simulink model "MPC_Extended_Plant_Simulink"  (R2024a)
settings: Solver=ode4  StartTime=0.0  StopTime=20  FixedStep=1e-3  RelTol=1e-3
values from neighbouring files (symbols this model uses):
  init =     [P1.mat]    (also in P2.mat; P3.mat)
  input =     [P1.mat]    (also in P2.mat; P3.mat)
  par =     [P1.mat]    (also in P2.mat; P3.mat)
  Ts = 0.01    [MPC_Extended_Plant.m]    (also in P1.mat; P2.mat; P3.mat)
  V_ref = 16.6666666667    [P1.mat]    (also in P2.mat; P3.mat)
undefined symbols (not defined in the file or in its folder): data
libraries: simulink x8
(part 1 of 2)
settings Model: Creator=bshyrokau  LastModifiedBy=lbsch
settings SolverCC: AlgebraicLoopSolver=TrustRegion
settings DataIOCC: SaveOutput=off  SignalLogging=off  DSMLogging=off  SaveTime=off  ReturnWorkspaceOutputs=off
settings OptimizationCC: ReuseModelBlockBuffer=off  LifeSpan=inf
settings DebuggingCC: UnconnectedInputMsg=warning  UnconnectedOutputMsg=warning  UnconnectedLineMsg=warning  AllowSymbolicDim=off  SFUnexpectedBacktrackingDiag=warning  SFNoUnconditionalDefaultTransitionDiag=warning  SFExecutionAtInitializationDiag=none  ArithmeticOperatorsInVariantConditions=warning
settings ModelReferenceCC: EnableRefExpFcnMdlSchedulingChecks=on  PropagateSignalLabelsOutOfModel=off
settings SFSimCC: SimUseLocalCustomCode=off  CustomCodeUndefinedFunction=UseInterfaceOnly
settings RTWCC: RTWUseLocalCustomCode=off  GPUComputeCapability=3.5  DLArmComputeVersion=19.05
settings CodeAppCC: StateflowObjectComments=on
settings GRTTargetCC: TargetLangStandard=C89/C90 (ANSI)
settings ConfigComp: CovMetricSettings=dw  CovSaveCumulativeToWorkspaceVar=on  CovSaveSingleToWorkspaceVar=on  CovExternalEMLEnable=off
settings SimscapeCC: SimscapeNormalizeSystem=off
settings ConfigurationSet: Description=SimMechanics 2G

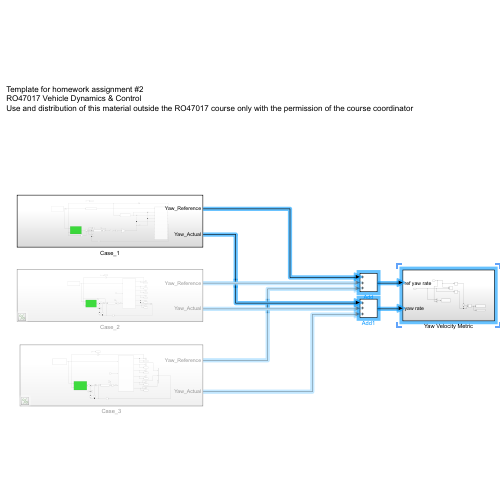
[thumbnail: Simulink's stored preview of the top-level diagram]
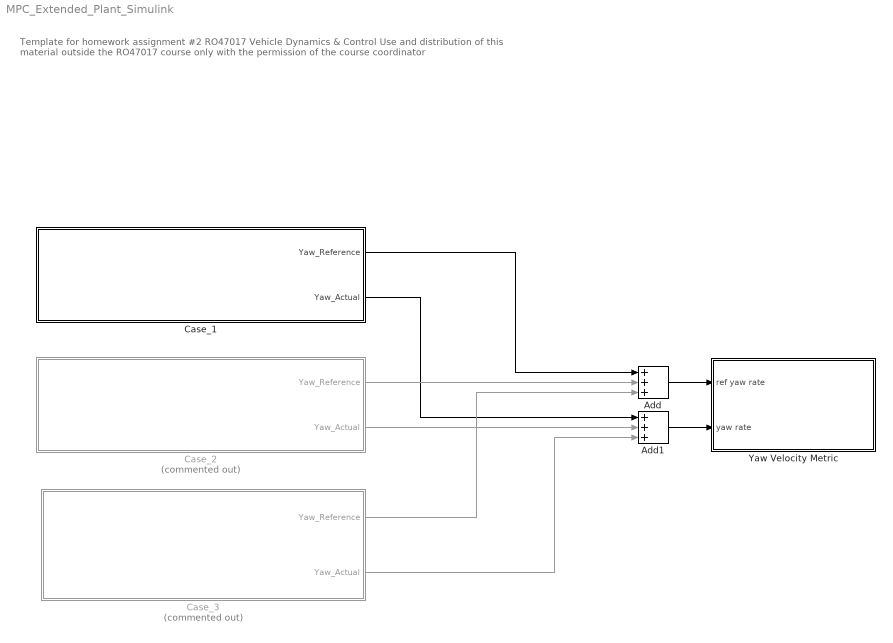
== system MPC_Extended_Plant_Simulink ==
  note: Template for homework assignment #2
      | RO47017 Vehicle Dynamics & Control
      | Use and distribution of this material outside the RO47017 course only with the permission of the course coordinator
  Add : Sum  Inputs=3
  Add1 : Sum  Inputs=3
  Case_1 : Subsystem
  Case_2 : Subsystem  Commented=on
  Case_3 : Subsystem  Commented=on
  Yaw Velocity Metric : Subsystem
  wires:
  Case_1/1(Yaw_Reference) -> Add/1
  Add/1 -> Yaw Velocity Metric/1(ref yaw rate)
  Case_1/2(Yaw_Actual) -> Add1/1
  Case_3/2(Yaw_Actual) -> Add1/3
  Case_3/1(Yaw_Reference) -> Add/3
  Case_2/2(Yaw_Actual) -> Add1/2
  Case_2/1(Yaw_Reference) -> Add/2
  Add1/1 -> Yaw Velocity Metric/2(yaw rate)

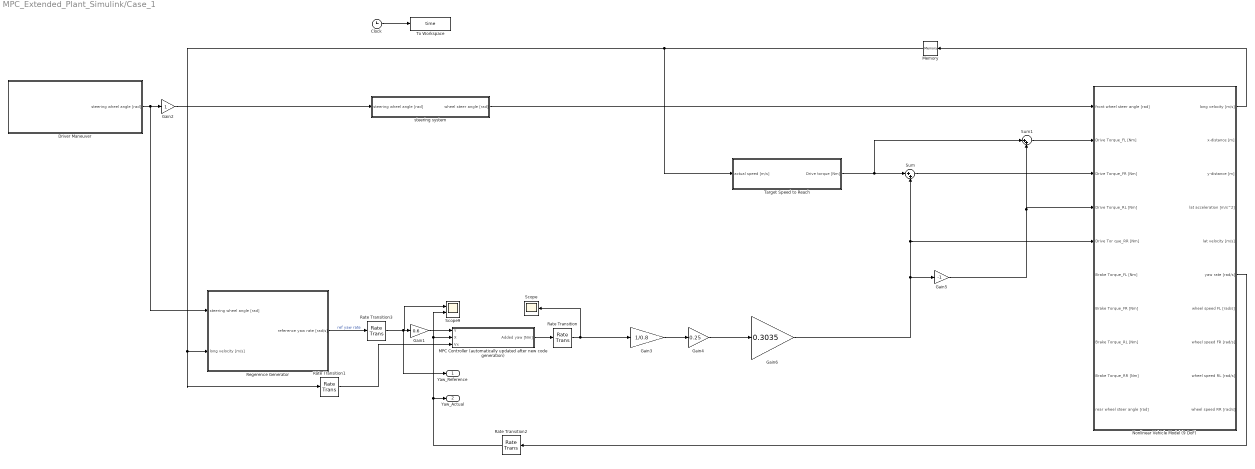
== system MPC_Extended_Plant_Simulink/Case_1 ==
  Clock : Clock
  Driver Maneuver : Subsystem
  Gain1 : Gain  Gain=0.6
  Gain2 : Gain
  Gain3 : Gain  Gain=1/0.8
  Gain4 : Gain  Gain=0.25
  Gain5 : Gain  Gain=-1
  Gain6 : Gain  Gain=0.3035
  MPC Controller (automatically updated after new code generation) : Subsystem
  Memory : Memory  InitialCondition=V_ref
  Nonlinear Vehicle Model (9 DoF) : Subsystem
      mask help: Simulink:masks:GenSFuncDesc_MD
      mask Help: eval('feval(''rtwprivate'',''rtwhelpview'',''rtw_sfcn_block'')');
  Rate Transition : RateTransition
  Rate Transition1 : RateTransition  InitialCondition=V_ref  OutPortSampleTime=Ts
  Rate Transition2 : RateTransition  OutPortSampleTime=Ts
  Rate Transition3 : RateTransition  OutPortSampleTime=Ts
  Regerence Generator : Subsystem
  Scope : Scope
  Scope9 : Scope  NumInputPorts=2
  Sum : Sum  Inputs=|++
  Sum1 : Sum  Inputs=|++
  Target Speed to Reach : Subsystem
  To Workspace : ToWorkspace  VariableName=time  SampleTime=-1
  steering system : Subsystem
  Yaw_Reference : Outport
  Yaw_Actual : Outport  Port=2
  wires:
  MPC Controller (automatically updated after new code generation)/1(Added yaw [Nm]) -> Rate Transition/1
  Gain1/1 -> MPC Controller (automatically updated after new code generation)/1(Y)
  Rate Transition2/1 -> Yaw_Actual/1, Scope9/2, MPC Controller (automatically updated after new code generation)/2(X)
  Rate Transition3/1 -> Yaw_Reference/1, Gain1/1, Scope9/1
  Clock/1 -> To Workspace/1
  Rate Transition1/1 -> MPC Controller (automatically updated after new code generation)/3(Vx)
  Rate Transition/1 -> Scope/1, Gain3/1
  Regerence Generator/1(reference yaw rate [rad/s]) -> Rate Transition3/1  "ref yaw rate"
  Driver Maneuver/1(steering wheel angle [rad]) -> Regerence Generator/1(steering wheel angle [rad]), Gain2/1
  Gain2/1 -> steering system/1(steering wheel angle [rad])
  steering system/1(wheel steer angle [rad]) -> Nonlinear Vehicle Model (9 DoF)/1(front wheel steer angle [rad])
  Gain6/1 -> Gain5/1, Nonlinear Vehicle Model (9 DoF)/5(Drive Tor	que_RR [Nm]), Sum/2
  Gain4/1 -> Gain6/1
  Gain3/1 -> Gain4/1
  Gain5/1 -> Nonlinear Vehicle Model (9 DoF)/4(Drive Torque_RL [Nm]), Sum1/2
  Nonlinear Vehicle Model (9 DoF)/6(yaw rate [rad/s]) -> Rate Transition2/1
  Sum/1 -> Nonlinear Vehicle Model (9 DoF)/3(Drive Torque_FR [Nm])
  Target Speed to Reach/1(Drive torque [Nm]) -> Sum1/1, Sum/1
  Sum1/1 -> Nonlinear Vehicle Model (9 DoF)/2(Drive Torque_FL [Nm])
  Memory/1 -> Rate Transition1/1, Regerence Generator/2(long velocity [m/s]), Target Speed to Reach/1(actual speed [m/s])
  Nonlinear Vehicle Model (9 DoF)/1(long velocity [m/s]) -> Memory/1

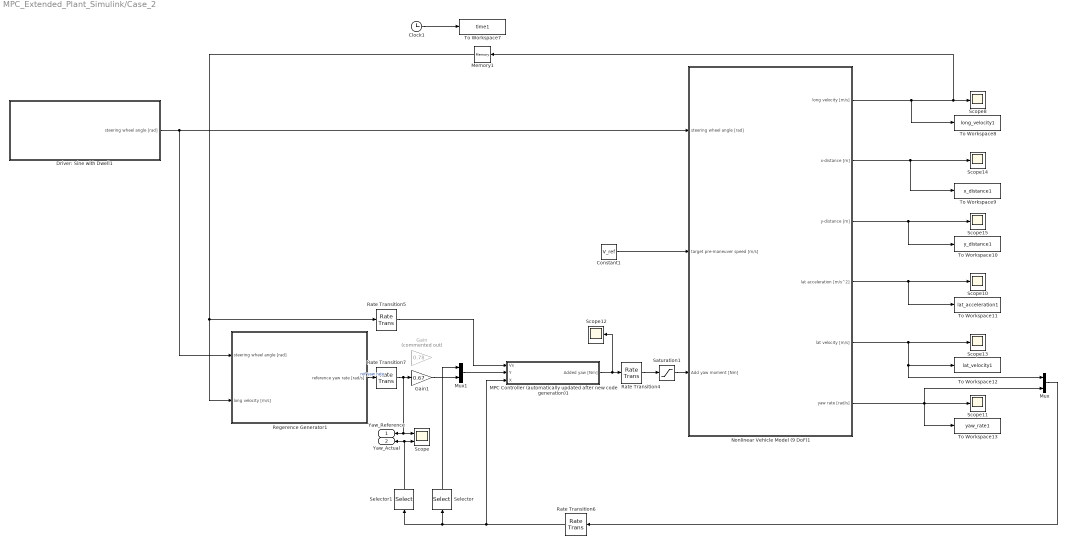
== system MPC_Extended_Plant_Simulink/Case_2 ==
  Clock1 : Clock
  Constant1 : Constant  Value=V_ref
  Driver: Sine with Dwell1 : Subsystem
  Gain : Gain  Commented=on  Gain=0.78
  Gain1 : Gain  Gain=0.67
  MPC Controller (automatically updated after new code generation)1 : Subsystem
  Memory1 : Memory  InitialCondition=V_ref
  Mux : Mux  Inputs=2
  Mux1 : Mux  Inputs=2
  Nonlinear Vehicle Model (9 DoF)1 : Subsystem
      mask help: Simulink:masks:GenSFuncDesc_MD
      mask Help: eval('feval(''rtwprivate'',''rtwhelpview'',''rtw_sfcn_block'')');
  Rate Transition4 : RateTransition
  Rate Transition5 : RateTransition  InitialCondition=V_ref  OutPortSampleTime=Ts
  Rate Transition6 : RateTransition  InitialCondition=[0 0]  OutPortSampleTime=Ts
  Rate Transition7 : RateTransition  OutPortSampleTime=Ts
  Regerence Generator1 : Subsystem
  Saturation1 : Saturate  UpperLimit=10000  LowerLimit=-10000
  Scope : Scope  NumInputPorts=2
  Scope{8,10..15} (7 alike) : Scope
  Selector : Selector  InputPortWidth=2  IndexOptions=Index vector (dialog)  Indices=1  OutputSizes=1
  Selector1 : Selector  InputPortWidth=2  IndexOptions=Index vector (dialog)  Indices=2  OutputSizes=1
  To Workspace10 : ToWorkspace  VariableName=y_distance1  SampleTime=-1
  To Workspace11 : ToWorkspace  VariableName=lat_acceleration1  SampleTime=-1
  To Workspace12 : ToWorkspace  VariableName=lat_velocity1  SampleTime=-1
  To Workspace13 : ToWorkspace  VariableName=yaw_rate1  SampleTime=-1
  To Workspace7 : ToWorkspace  VariableName=time1  SampleTime=-1
  To Workspace8 : ToWorkspace  VariableName=long_velocity1  SampleTime=-1
  To Workspace9 : ToWorkspace  VariableName=x_distance1  SampleTime=-1
  Yaw_Reference : Outport
  Yaw_Actual : Outport  Port=2
  wires:
  Rate Transition4/1 -> Saturation1/1
  Nonlinear Vehicle Model (9 DoF)1/3(y-distance [m]) -> To Workspace10/1, Scope15/1
  MPC Controller (automatically updated after new code generation)1/1(Added yaw [Nm]) -> Scope12/1, Rate Transition4/1
  Constant1/1 -> Nonlinear Vehicle Model (9 DoF)1/2(target pre-maneuver speed [m/s])
  Rate Transition6/1 -> Selector1/1, Selector/1, MPC Controller (automatically updated after new code generation)1/3(X)
  Rate Transition5/1 -> MPC Controller (automatically updated after new code generation)1/1(Vx)
  Nonlinear Vehicle Model (9 DoF)1/2(x-distance [m]) -> To Workspace9/1, Scope14/1
  Mux/1 -> Rate Transition6/1
  Saturation1/1 -> Nonlinear Vehicle Model (9 DoF)1/3(Add yaw moment [Nm])
  Nonlinear Vehicle Model (9 DoF)1/1(long velocity [m/s]) -> To Workspace8/1, Memory1/1, Scope8/1
  Regerence Generator1/1(reference yaw rate [rad/s]) -> Rate Transition7/1  "ref yaw rate"
  Memory1/1 -> Regerence Generator1/2(long velocity [m/s]), Rate Transition5/1
  Driver: Sine with Dwell1/1(steering wheel angle [rad]) -> Regerence Generator1/1(steering wheel angle [rad]), Nonlinear Vehicle Model (9 DoF)1/1(steering wheel angle [rad])
  Nonlinear Vehicle Model (9 DoF)1/6(yaw rate [rad/s]) -> Mux/2, Scope11/1, To Workspace13/1
  Clock1/1 -> To Workspace7/1
  Nonlinear Vehicle Model (9 DoF)1/4(lat acceleration [m/s^2]) -> To Workspace11/1, Scope10/1
  Nonlinear Vehicle Model (9 DoF)1/5(lat velocity [m/s]) -> Mux/1, To Workspace12/1, Scope13/1
  Mux1/1 -> MPC Controller (automatically updated after new code generation)1/2(Y)
  Selector1/1 -> Scope/2, Yaw_Actual/1
  Gain1/1 -> Mux1/2
  Rate Transition7/1 -> Yaw_Reference/1, Scope/1, Gain1/1
  Selector/1 -> Mux1/1

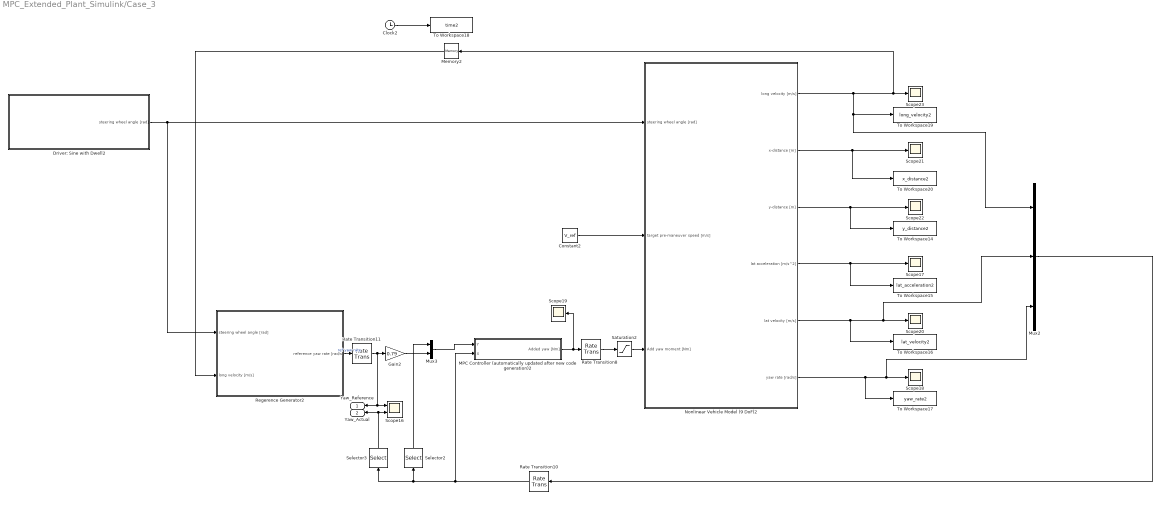
== system MPC_Extended_Plant_Simulink/Case_3 ==
  Clock2 : Clock
  Constant2 : Constant  Value=V_ref
  Driver: Sine with Dwell2 : Subsystem
  Gain2 : Gain  Gain=0.79
  MPC Controller (automatically updated after new code generation)2 : Subsystem
  Memory2 : Memory  InitialCondition=V_ref
  Mux2 : Mux  Inputs=3
  Mux3 : Mux  Inputs=2
  Nonlinear Vehicle Model (9 DoF)2 : Subsystem
      mask help: Simulink:masks:GenSFuncDesc_MD
      mask Help: eval('feval(''rtwprivate'',''rtwhelpview'',''rtw_sfcn_block'')');
  Rate Transition10 : RateTransition  InitialCondition=[V_ref 0 0]  OutPortSampleTime=Ts
  Rate Transition11 : RateTransition  OutPortSampleTime=Ts
  Rate Transition8 : RateTransition
  Regerence Generator2 : Subsystem
  Saturation2 : Saturate  UpperLimit=10000  LowerLimit=-10000
  Scope16 : Scope  NumInputPorts=2
  Scope{17..23} (7 alike) : Scope
  Selector2 : Selector  InputPortWidth=3  IndexOptions=Index vector (dialog)  Indices=[1 2]  OutputSizes=1
  Selector3 : Selector  InputPortWidth=3  IndexOptions=Index vector (dialog)  Indices=3  OutputSizes=1
  To Workspace14 : ToWorkspace  VariableName=y_distance2  SampleTime=-1
  To Workspace15 : ToWorkspace  VariableName=lat_acceleration2  SampleTime=-1
  To Workspace16 : ToWorkspace  VariableName=lat_velocity2  SampleTime=-1
  To Workspace17 : ToWorkspace  VariableName=yaw_rate2  SampleTime=-1
  To Workspace18 : ToWorkspace  VariableName=time2  SampleTime=-1
  To Workspace19 : ToWorkspace  VariableName=long_velocity2  SampleTime=-1
  To Workspace20 : ToWorkspace  VariableName=x_distance2  SampleTime=-1
  Yaw_Reference : Outport
  Yaw_Actual : Outport  Port=2
  wires:
  Nonlinear Vehicle Model (9 DoF)2/6(yaw rate [rad/s]) -> Mux2/3, Scope18/1, To Workspace17/1
  Rate Transition10/1 -> Selector3/1, Selector2/1, MPC Controller (automatically updated after new code generation)2/2(X)
  Driver: Sine with Dwell2/1(steering wheel angle [rad]) -> Regerence Generator2/1(steering wheel angle [rad]), Nonlinear Vehicle Model (9 DoF)2/1(steering wheel angle [rad])
  Nonlinear Vehicle Model (9 DoF)2/1(long velocity [m/s]) -> Mux2/1, To Workspace19/1, Memory2/1, Scope23/1
  Nonlinear Vehicle Model (9 DoF)2/5(lat velocity [m/s]) -> To Workspace16/1, Mux2/2, Scope20/1
  Nonlinear Vehicle Model (9 DoF)2/2(x-distance [m]) -> To Workspace20/1, Scope21/1
  Nonlinear Vehicle Model (9 DoF)2/4(lat acceleration [m/s^2]) -> To Workspace15/1, Scope17/1
  MPC Controller (automatically updated after new code generation)2/1(Added yaw [Nm]) -> Scope19/1, Rate Transition8/1
  Mux3/1 -> MPC Controller (automatically updated after new code generation)2/1(Y)
  Mux2/1 -> Rate Transition10/1
  Nonlinear Vehicle Model (9 DoF)2/3(y-distance [m]) -> To Workspace14/1, Scope22/1
  Memory2/1 -> Regerence Generator2/2(long velocity [m/s])
  Selector3/1 -> Scope16/2, Yaw_Actual/1
  Regerence Generator2/1(reference yaw rate [rad/s]) -> Rate Transition11/1  "ref yaw rate"
  Rate Transition11/1 -> Yaw_Reference/1, Scope16/1, Gain2/1
  Saturation2/1 -> Nonlinear Vehicle Model (9 DoF)2/3(Add yaw moment [Nm])
  Clock2/1 -> To Workspace18/1
  Rate Transition8/1 -> Saturation2/1
  Constant2/1 -> Nonlinear Vehicle Model (9 DoF)2/2(target pre-maneuver speed [m/s])
  Gain2/1 -> Mux3/2
  Selector2/1 -> Mux3/1

== system MPC_Extended_Plant_Simulink/Yaw Velocity Metric ==
  ref yaw rate : Inport
  yaw rate : Inport  Port=2
  Display2 : Display
  Divide : Product  Inputs=*/
  Integrator : Integrator  InitialCondition=0.000001
  Integrator1 : Integrator
  Mux : Mux  Inputs=2
  Scope10 : Scope  NumInputPorts=2
  Sum : Sum  Inputs=+-
  To Workspace1 : ToWorkspace  VariableName=yaw_results  SaveFormat=Timeseries  SampleTime=-1
  To Workspace10 : ToWorkspace  VariableName=yaw_velocity_metric  SampleTime=-1
      settings: MaxDataPoints=1
  wires:
  yaw rate/1 -> Mux/2, Scope10/1, Integrator1/1
  ref yaw rate/1 -> Mux/1, Integrator/1, Scope10/2
  Divide/1 -> To Workspace10/1, Display2/1
  Integrator/1 -> Sum/2, Divide/2
  Integrator1/1 -> Sum/1
  Sum/1 -> Divide/1
  Mux/1 -> To Workspace1/1

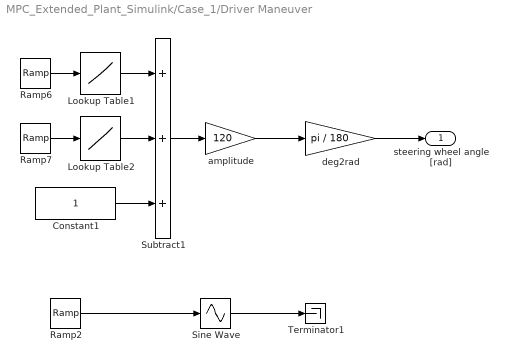
== system MPC_Extended_Plant_Simulink/Case_1/Driver Maneuver ==
  Constant1 : Constant
  Lookup Table1 : Lookup  InputValues=[0:0.1:3*pi/2 3*pi/2+eps]*0.7  Table=sin([0:0.1:3*pi/2 3*pi/2+eps])  LookUpMeth=Interpolation-Use End Values  SaturateOnIntegerOverflow=off
  Lookup Table2 : Lookup  InputValues=[3*pi/2:0.1:2*pi 2*pi+eps]*0.7  Table=sin([3*pi/2:0.1:2*pi 2*pi+eps])  LookUpMeth=Interpolation-Use End Values  SaturateOnIntegerOverflow=off
  Ramp2 : simulink/Sources/Ramp  slope=1  start=10  InitialOutput=0
  Ramp6 : simulink/Sources/Ramp  slope=pi  start=10  InitialOutput=0
  Ramp7 : simulink/Sources/Ramp  slope=pi  start=10+0.5  InitialOutput=0
  Sine Wave : Sin  TimeSource=Use external signal  Amplitude=30/180*pi  Frequency=2*pi*0.2  SampleTime=0
  Subtract1 : Sum  Inputs=+++
  Terminator1 : Terminator
  amplitude : Gain  Gain=120
  deg2rad : Gain  Gain=pi / 180
  steering wheel angle [rad] : Outport  VectorParamsAs1DForOutWhenUnconnected=off
  wires:
  Ramp6/1 -> Lookup Table1/1
  Ramp7/1 -> Lookup Table2/1
  Lookup Table2/1 -> Subtract1/2
  Lookup Table1/1 -> Subtract1/1
  Constant1/1 -> Subtract1/3
  Subtract1/1 -> amplitude/1
  amplitude/1 -> deg2rad/1
  Ramp2/1 -> Sine Wave/1
  deg2rad/1 -> steering wheel angle [rad]/1
  Sine Wave/1 -> Terminator1/1

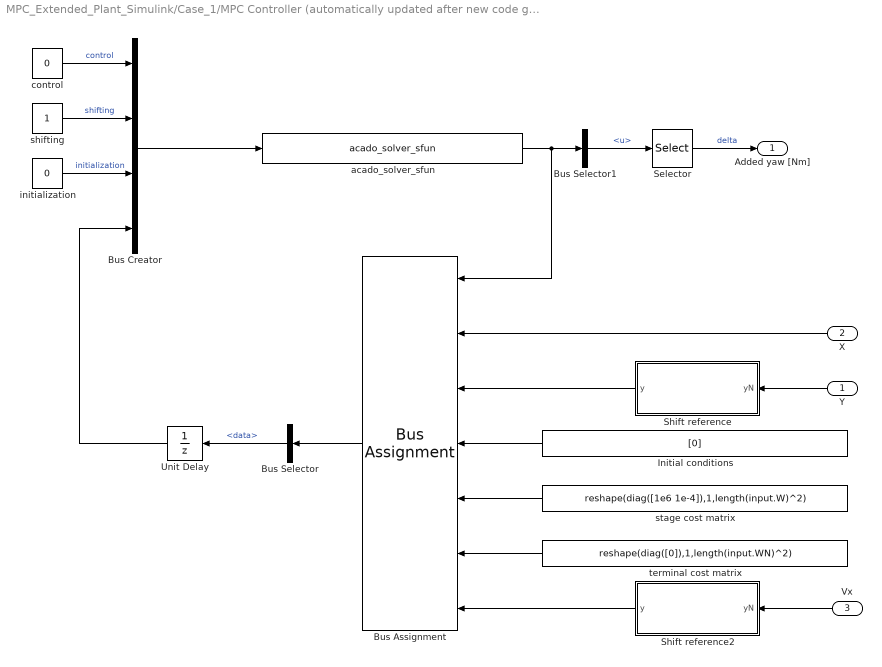
== system MPC_Extended_Plant_Simulink/Case_1/MPC Controller (automatically updated after new code generation) ==
  Y : Inport
  X : Inport  Port=2
  Vx : Inport  Port=3
  Bus Assignment : BusAssignment  AssignedSignals=data.x0,data.y,data.yN,data.W,data.WN,data.od
  Bus Creator : BusCreator  Inputs=4  OutDataTypeStr=Bus: ACADOinput
  Bus Selector : BusSelector  OutputSignals=data
  Bus Selector1 : BusSelector  OutputSignals=data.u
  Initial conditions : Constant  Value=[0]
  Selector : Selector  InputPortWidth=Np  IndexOptions=Starting index (dialog)  Indices=[1]  OutputSizes=1
  Shift reference : MATLAB Function  TreatAsAtomicUnit=on
  Shift reference2 : MATLAB Function  TreatAsAtomicUnit=on
  Unit Delay : UnitDelay  InitialCondition=init  SampleTime=Ts  HasFrameUpgradeWarning=on
  acado_solver_sfun : S-Function  FunctionName=acado_solver_sfun  SFunctionDeploymentMode=off  EnableBusSupport=off  mask(Legacy Function){SFunctionSpec=acado_step(ACADOinput u1[1], ACADOoutput y1[1]), ShowSpec=on}
      mask prompts: ShowSpec "Display function specification"
      mask help:
      | This block allows you to call the legacy functions specified by the following Legacy Code Tool definition:
      | def.SFunctionName = 'acado_solver_sfun';
      | def.OutputFcnSpec = 'acado_step(ACADOinput u1[1], ACADOoutput y1[1])';
      | def.StartFcnSpec = 'acado_initialize( void )';
      | def.TerminateFcnSpec = 'acado_cleanup( void )';
      | def.HeaderFiles = {'acado_common.h', 'acado_solver_sfunction.h'};
      | def.SourceFiles = {'acado_solver.c', 'acado_integrator.c', 'acado_auxiliary_functions.c', 'acado_solver_sfunction.c', 'acado_qpoases3_interface.c', 'qpoases3\src\Bounds.c', 'qpoases3\src\Constraints.c', 'qpoases3\src\Indexlist.c', 'qpoases3\src\Matrices.c', 'qpoases3\src\MessageHandling.c', 'qpoases3\src\Options.c', 'qpoases3\src\Flipper.c', 'qpoases3\src\QProblem.c', 'qpoases3\src\QProblemB.c', 'qpoases3\src\Utils.c'};
      mask Help: <p>This block was generated automatically by the Legacy Code Tool. For detailed help on this tool, call<a href="matlab:legacy_code('help')"> legacy_code('help')</a>.</p>
      mask Callback ShowSpec:
      | if strcmp(get_param(gcbh, 'ShowSpec'), 'on')
      |   set_param(gcbh, 'MaskDisplay', sprintf('fprintf(''%s'');', get_param(gcbh, 'SFunctionSpec')));
      | else
      |   set_param(gcbh, 'MaskDisplay', sprintf('fprintf(''%s'');', get_param(gcbh, 'FunctionName')));
      | end
      mask Display: fprintf('acado_step(ACADOinput u1[1], ACADOoutput y1[1])');
  control : Constant  Value=0  OutDataTypeStr=int32
  initialization : Constant  Value=0  OutDataTypeStr=int32
  shifting : Constant  OutDataTypeStr=int32
  stage cost matrix : Constant  Value=reshape(diag([1e6 1e-4]),1,length(input.W)^2)
  terminal cost matrix : Constant  Value=reshape(diag([0]),1,length(input.WN)^2)
  Added yaw [Nm] : Outport
  wires:
  control/1 -> Bus Creator/1  "control"
  Bus Selector1/1 -> Selector/1  "<u>"
  initialization/1 -> Bus Creator/3  "initialization"
  acado_solver_sfun/1 -> Bus Selector1/1, Bus Assignment/1
  shifting/1 -> Bus Creator/2  "shifting"
  Bus Assignment/1 -> Bus Selector/1
  terminal cost matrix/1 -> Bus Assignment/6
  Initial conditions/1 -> Bus Assignment/4
  Shift reference/1(y) -> Bus Assignment/3
  stage cost matrix/1 -> Bus Assignment/5
  Bus Selector/1 -> Unit Delay/1  "<data>"
  Unit Delay/1 -> Bus Creator/4
  Bus Creator/1 -> acado_solver_sfun/1
  Selector/1 -> Added yaw [Nm]/1  "delta"
  Y/1 -> Shift reference/1(yN)
  X/1 -> Bus Assignment/2
  Shift reference2/1(y) -> Bus Assignment/7
  Vx/1 -> Shift reference2/1(yN)

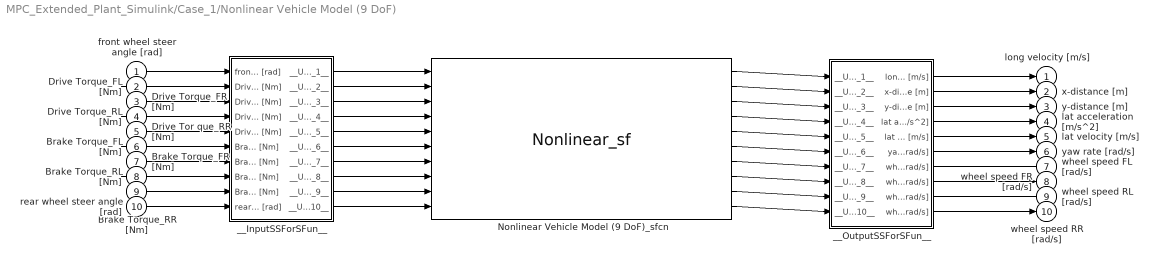
== system MPC_Extended_Plant_Simulink/Case_1/Nonlinear Vehicle Model (9 DoF) ==
  front wheel steer angle [rad] : Inport
  Drive Torque_FL [Nm] : Inport  Port=2
  Drive Torque_FR [Nm] : Inport  Port=3
  Drive Torque_RL [Nm] : Inport  Port=4
  Drive Tor	que_RR [Nm] : Inport  Port=5
  Brake Torque_FL [Nm] : Inport  Port=6
  Brake Torque_FR [Nm] : Inport  Port=7
  Brake Torque_RL [Nm] : Inport  Port=8
  Brake Torque_RR [Nm] : Inport  Port=9
  rear wheel steer angle [rad] : Inport  Port=10
  Nonlinear Vehicle Model (9 DoF)_sfcn : S-Function  FunctionName=Nonlinear_sf  SFunctionModules=""  SFunctionDeploymentMode=off  EnableBusSupport=off  mask{rtw_sf_name=Nonlinear_sf, showVar=off}
      mask prompts: rtw_sf_name "Simulink:masks:GenSFuncName_MP"; showVar "Simulink:masks:GenSFuncShowModuleList_MP"
      mask help: Simulink:masks:GenSFuncDesc_MD
      mask init:
      | displist = '';
      | if ~strcmp(get_param(gcb, 'FunctionName'), rtw_sf_name);
      |   set_param(gcb, 'FunctionName', rtw_sf_name);
      | end
      | % Check if we are generating code
      | rtw_mode = false;
      | if strcmpi(get_param(bdroot(gcb),'SimulationStatus'),'Initializing')
      | 	rtw_mode = strcmpi(get_param(bdroot(gcb),'BuildingRTWCode'),'on') && ...
      | 		~strcmpi(get_param(bdroot(gcb),'TargetStyle'),'SimulationTarget');
      | end
      | if showVar || rtw_mode
      | 	if exist('rtwsfunc') == 2 | exist('rtwsfunc') == 6
      | 		tmplist = rtwsfunc(rtw_sf_name,gcb);
      | 		tmplist = DAStudio.message('Simulink:masks:GenSFuncListOfModules_IC', tmplist);
      | 	elseif showVar
      | 		tmplist1 = DAStudio.message('Simulink:masks:GenSFuncListOfModules_IC', '');
      |         tmplist2 = DAStudio.message('Simulink:masks:GenSFuncNotLicensed_IC');
      |         tmplist = [tmplist1 tmplist2];
      |  	end
      | end
      | if showVar
      |   displist = tmplist;
      | end
      settings: CopyFcn=|
      | if ~strcmp(get_param(gcb,'Linkstatus'),'none') && ...
      | ~strcmp(get_param(gcb,'Linkstatus'),'implicit')
      |   set_param(gcb,'LinkStatus','none');
      | end
      mask Help: eval('feval(''rtwprivate'',''rtwhelpview'',''rtw_sfcn_block'')');
      mask Display:
      | port_label('input',1,'front wheel steer angle [rad]');
      | port_label('input',2,'Drive Torque_FL [Nm]');
      | port_label('input',3,'Drive Torque_FR [Nm]');
      | port_label('input',4,'Drive Torque_RL [Nm]');
      | port_label('input',5,'Drive Tor	que_RR [Nm]');
      | port_label('input',6,'Brake Torque_FL [Nm]');
      | port_label('input',7,'Brake Torque_FR [Nm]');
      | port_label('input',8,'Brake Torque_RL [Nm]');
      | port_label('input',9,'Brake Torque_RR [Nm]');
      | port_label('input',10,'rear wheel steer angle [rad]');
      | port_label('output',1,'long velocity [m/s]');
      | port_label('output',2,'x-distance [m]');
      | port_label('output',3,'y-distance [m]');
      | port_label('output',4,'lat acceleration [m/s^2]');
      | port_label('output',5,'lat velocity [m/s]');
      | port_label('output',6,'yaw rate [rad/s]');
      | port_label('output',7,'wheel speed FL [rad/s]');
      | port_label('output',8,'wheel speed FR [rad/s]');
      | port_label('output',9,'wheel speed RL [rad/s]');
      | port_label('output',10,'wheel speed RR [rad/s]');
  __InputSSForSFun__ : Subsystem
  __OutputSSForSFun__ : Subsystem
  long velocity [m/s] : Outport  VectorParamsAs1DForOutWhenUnconnected=off
  x-distance [m] : Outport  Port=2  VectorParamsAs1DForOutWhenUnconnected=off
  y-distance [m] : Outport  Port=3  VectorParamsAs1DForOutWhenUnconnected=off
  lat acceleration [m/s^2] : Outport  Port=4  VectorParamsAs1DForOutWhenUnconnected=off
  lat velocity [m/s] : Outport  Port=5  VectorParamsAs1DForOutWhenUnconnected=off
  yaw rate [rad/s] : Outport  Port=6  VectorParamsAs1DForOutWhenUnconnected=off
  wheel speed FL [rad/s] : Outport  Port=7  VectorParamsAs1DForOutWhenUnconnected=off
  wheel speed FR [rad/s] : Outport  Port=8  VectorParamsAs1DForOutWhenUnconnected=off
  wheel speed RL [rad/s] : Outport  Port=9  VectorParamsAs1DForOutWhenUnconnected=off
  wheel speed RR [rad/s] : Outport  Port=10  VectorParamsAs1DForOutWhenUnconnected=off
  wires:
  front wheel steer angle [rad]/1 -> __InputSSForSFun__/1(front wheel steer angle [rad])
  Drive Torque_FL [Nm]/1 -> __InputSSForSFun__/2(Drive Torque_FL [Nm])
  Drive Torque_FR [Nm]/1 -> __InputSSForSFun__/3(Drive Torque_FR [Nm])
  Drive Torque_RL [Nm]/1 -> __InputSSForSFun__/4(Drive Torque_RL [Nm])
  Drive Tor	que_RR [Nm]/1 -> __InputSSForSFun__/5(Drive Tor	que_RR [Nm])
  Brake Torque_FL [Nm]/1 -> __InputSSForSFun__/6(Brake Torque_FL [Nm])
  Brake Torque_FR [Nm]/1 -> __InputSSForSFun__/7(Brake Torque_FR [Nm])
  Brake Torque_RL [Nm]/1 -> __InputSSForSFun__/8(Brake Torque_RL [Nm])
  Brake Torque_RR [Nm]/1 -> __InputSSForSFun__/9(Brake Torque_RR [Nm])
  rear wheel steer angle [rad]/1 -> __InputSSForSFun__/10(rear wheel steer angle [rad])
  __InputSSForSFun__/1(__UniqueOutportName__1__) -> Nonlinear Vehicle Model (9 DoF)_sfcn/1
  __InputSSForSFun__/2(__UniqueOutportName__2__) -> Nonlinear Vehicle Model (9 DoF)_sfcn/2
  __InputSSForSFun__/3(__UniqueOutportName__3__) -> Nonlinear Vehicle Model (9 DoF)_sfcn/3
  __InputSSForSFun__/4(__UniqueOutportName__4__) -> Nonlinear Vehicle Model (9 DoF)_sfcn/4
  __InputSSForSFun__/5(__UniqueOutportName__5__) -> Nonlinear Vehicle Model (9 DoF)_sfcn/5
  __InputSSForSFun__/6(__UniqueOutportName__6__) -> Nonlinear Vehicle Model (9 DoF)_sfcn/6
  __InputSSForSFun__/7(__UniqueOutportName__7__) -> Nonlinear Vehicle Model (9 DoF)_sfcn/7
  __InputSSForSFun__/8(__UniqueOutportName__8__) -> Nonlinear Vehicle Model (9 DoF)_sfcn/8
  __InputSSForSFun__/9(__UniqueOutportName__9__) -> Nonlinear Vehicle Model (9 DoF)_sfcn/9
  __InputSSForSFun__/10(__UniqueOutportName__10__) -> Nonlinear Vehicle Model (9 DoF)_sfcn/10
  Nonlinear Vehicle Model (9 DoF)_sfcn/1 -> __OutputSSForSFun__/1(__UniqueInportName__1__)
  Nonlinear Vehicle Model (9 DoF)_sfcn/2 -> __OutputSSForSFun__/2(__UniqueInportName__2__)
  Nonlinear Vehicle Model (9 DoF)_sfcn/3 -> __OutputSSForSFun__/3(__UniqueInportName__3__)
  Nonlinear Vehicle Model (9 DoF)_sfcn/4 -> __OutputSSForSFun__/4(__UniqueInportName__4__)
  Nonlinear Vehicle Model (9 DoF)_sfcn/5 -> __OutputSSForSFun__/5(__UniqueInportName__5__)
  Nonlinear Vehicle Model (9 DoF)_sfcn/6 -> __OutputSSForSFun__/6(__UniqueInportName__6__)
  Nonlinear Vehicle Model (9 DoF)_sfcn/7 -> __OutputSSForSFun__/7(__UniqueInportName__7__)
  Nonlinear Vehicle Model (9 DoF)_sfcn/8 -> __OutputSSForSFun__/8(__UniqueInportName__8__)
  Nonlinear Vehicle Model (9 DoF)_sfcn/9 -> __OutputSSForSFun__/9(__UniqueInportName__9__)
  Nonlinear Vehicle Model (9 DoF)_sfcn/10 -> __OutputSSForSFun__/10(__UniqueInportName__10__)
  __OutputSSForSFun__/1(long velocity [m/s]) -> long velocity [m/s]/1
  __OutputSSForSFun__/2(x-distance [m]) -> x-distance [m]/1
  __OutputSSForSFun__/3(y-distance [m]) -> y-distance [m]/1
  __OutputSSForSFun__/4(lat acceleration [m/s^2]) -> lat acceleration [m/s^2]/1
  __OutputSSForSFun__/5(lat velocity [m/s]) -> lat velocity [m/s]/1
  __OutputSSForSFun__/6(yaw rate [rad/s]) -> yaw rate [rad/s]/1
  __OutputSSForSFun__/7(wheel speed FL [rad/s]) -> wheel speed FL [rad/s]/1
  __OutputSSForSFun__/8(wheel speed FR [rad/s]) -> wheel speed FR [rad/s]/1
  __OutputSSForSFun__/9(wheel speed RL [rad/s]) -> wheel speed RL [rad/s]/1
  __OutputSSForSFun__/10(wheel speed RR [rad/s]) -> wheel speed RR [rad/s]/1

== system MPC_Extended_Plant_Simulink/Case_1/Regerence Generator ==
  note: yawr_ref
  note: nonlinear response
  note: delta
  note: u
  steering wheel angle [rad] : Inport
  long velocity [m/s] : Inport  Port=2
  MATLAB Function : MATLAB Function  TreatAsAtomicUnit=on
  MATLAB Function1 : MATLAB Function  TreatAsAtomicUnit=on
  Transfer Fcn : TransferFcn  Numerator=[par.wn^2*par.tau par.wn^2]  Denominator=[1 2*par.kseta*par.wn par.wn^2]
  steering ratio : Gain  Gain=1/ par.i_steer
  reference yaw rate [rad/s] : Outport  VectorParamsAs1DForOutWhenUnconnected=off
  wires:
  steering wheel angle [rad]/1 -> steering ratio/1
  steering ratio/1 -> MATLAB Function/1(delta)
  long velocity [m/s]/1 -> MATLAB Function1/2(u), MATLAB Function/2(u)
  MATLAB Function/1(yawr_ss) -> MATLAB Function1/1(yawr_ss)
  MATLAB Function1/1(yawr_sat) -> Transfer Fcn/1
  Transfer Fcn/1 -> reference yaw rate [rad/s]/1

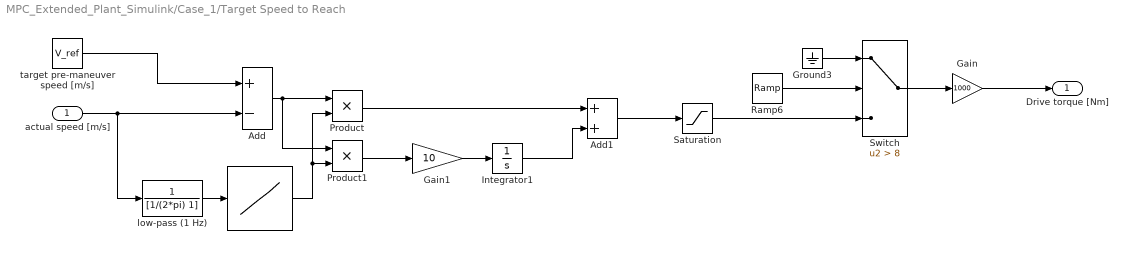
== system MPC_Extended_Plant_Simulink/Case_1/Target Speed to Reach ==
  actual speed [m/s] : Inport
  " " : Lookup_n-D  NumberOfTableDimensions=1  BreakpointsForDimension1="[-10  0  10 30]"  IndexSearchMethod=Linear search  Table=[0.1 0.1 1 1]  ExtrapMethod=Clip  RemoveProtectionInput=on  UseLastTableValue=on  RndMeth=Simplest
  Add : Sum  Inputs=+-
  Add1 : Sum
  Gain : Gain  Gain=1000
  Gain1 : Gain  Gain=10
  Ground3 : Ground
  Integrator1 : Integrator  LimitOutput=on  UpperSaturationLimit=0.1  LowerSaturationLimit=-0.1
  Product : Product  RndMeth=Zero
  Product1 : Product  RndMeth=Zero
  Ramp6 : simulink/Sources/Ramp  slope=1  start=0  InitialOutput=0
  Saturation : Saturate  UpperLimit=1  LowerLimit=0
  Switch : Switch  Criteria=u2 > Threshold  Threshold=8  SaturateOnIntegerOverflow=off  InputSameDT=off
  low-pass (1 Hz) : TransferFcn  Denominator=[1/(2*pi) 1]
  "target pre-maneuver speed [m/s] " : Constant  Value=V_ref
  Drive torque [Nm] : Outport
  wires:
  actual speed [m/s]/1 -> low-pass (1 Hz)/1, Add/2
  "target pre-maneuver speed [m/s] "/1 -> Add/1
  Gain1/1 -> Integrator1/1
  Product/1 -> Add1/1
  Add/1 -> Product/1, Product1/1
  Product1/1 -> Gain1/1
  " "/1 -> Product1/2, Product/2
  low-pass (1 Hz)/1 -> " "/1
  Add1/1 -> Saturation/1
  Integrator1/1 -> Add1/2
  Ramp6/1 -> Switch/2
  Switch/1 -> Gain/1
  Ground3/1 -> Switch/1
  Saturation/1 -> Switch/3
  Gain/1 -> Drive torque [Nm]/1

== system MPC_Extended_Plant_Simulink/Case_1/steering system ==
  steering wheel angle [rad] : Inport
  Delay : TransportDelay  DelayTime=par.teta_ss
  Steering Dynamics : TransferFcn  Numerator=[par.wn_ss^2]  Denominator=[1 2*par.zeta_ss*par.wn_ss par.wn_ss^2]
  steering ratio : Gain  Gain=1/ par.i_steer
  wheel steer angle [rad] : Outport  VectorParamsAs1DForOutWhenUnconnected=off
  wires:
  steering wheel angle [rad]/1 -> steering ratio/1
  Delay/1 -> Steering Dynamics/1
  steering ratio/1 -> Delay/1
  Steering Dynamics/1 -> wheel steer angle [rad]/1

== system MPC_Extended_Plant_Simulink/Case_2/Driver: Sine with Dwell1 ==
  Constant1 : Constant
  Lookup Table1 : Lookup  InputValues=[0:0.1:3*pi/2 3*pi/2+eps]*0.7  Table=sin([0:0.1:3*pi/2 3*pi/2+eps])  LookUpMeth=Interpolation-Use End Values  SaturateOnIntegerOverflow=off
  Lookup Table2 : Lookup  InputValues=[3*pi/2:0.1:2*pi 2*pi+eps]*0.7  Table=sin([3*pi/2:0.1:2*pi 2*pi+eps])  LookUpMeth=Interpolation-Use End Values  SaturateOnIntegerOverflow=off
  Ramp6 : simulink/Sources/Ramp  slope=pi  start=10  InitialOutput=0
  Ramp7 : simulink/Sources/Ramp  slope=pi  start=10+0.5  InitialOutput=0
  Subtract1 : Sum  Inputs=+++
  amplitude : Gain  Gain=120
  deg2rad : Gain  Gain=pi / 180
  steering wheel angle [rad] : Outport  VectorParamsAs1DForOutWhenUnconnected=off
  wires:
  Ramp6/1 -> Lookup Table1/1
  Ramp7/1 -> Lookup Table2/1
  Lookup Table2/1 -> Subtract1/2
  Lookup Table1/1 -> Subtract1/1
  Constant1/1 -> Subtract1/3
  Subtract1/1 -> amplitude/1
  amplitude/1 -> deg2rad/1
  deg2rad/1 -> steering wheel angle [rad]/1

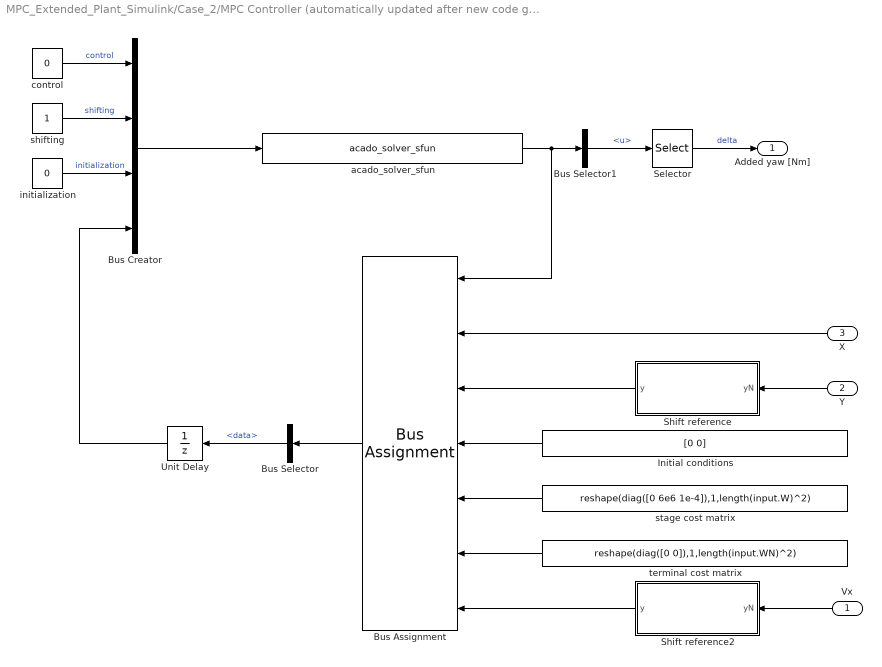
== system MPC_Extended_Plant_Simulink/Case_2/MPC Controller (automatically updated after new code generation)1 ==
  Vx : Inport
  Y : Inport  Port=2
  X : Inport  Port=3
  Bus Assignment : BusAssignment  AssignedSignals=data.x0,data.y,data.yN,data.W,data.WN,data.od
  Bus Creator : BusCreator  Inputs=4  OutDataTypeStr=Bus: ACADOinput
  Bus Selector : BusSelector  OutputSignals=data
  Bus Selector1 : BusSelector  OutputSignals=data.u
  Initial conditions : Constant  Value=[0 0]
  Selector : Selector  InputPortWidth=Np  IndexOptions=Starting index (dialog)  Indices=[1]  OutputSizes=1
  Shift reference : MATLAB Function  TreatAsAtomicUnit=on
  Shift reference2 : MATLAB Function  TreatAsAtomicUnit=on
  Unit Delay : UnitDelay  InitialCondition=init  SampleTime=Ts  HasFrameUpgradeWarning=on
  acado_solver_sfun : S-Function  FunctionName=acado_solver_sfun  SFunctionDeploymentMode=off  EnableBusSupport=off  mask(Legacy Function){SFunctionSpec=acado_step(ACADOinput u1[1], ACADOoutput y1[1]), ShowSpec=on}
      mask prompts: ShowSpec "Display function specification"
      mask help:
      | This block allows you to call the legacy functions specified by the following Legacy Code Tool definition:
      | def.SFunctionName = 'acado_solver_sfun';
      | def.OutputFcnSpec = 'acado_step(ACADOinput u1[1], ACADOoutput y1[1])';
      | def.StartFcnSpec = 'acado_initialize( void )';
      | def.TerminateFcnSpec = 'acado_cleanup( void )';
      | def.HeaderFiles = {'acado_common.h', 'acado_solver_sfunction.h'};
      | def.SourceFiles = {'acado_solver.c', 'acado_integrator.c', 'acado_auxiliary_functions.c', 'acado_solver_sfunction.c', 'acado_qpoases3_interface.c', 'qpoases3\src\Bounds.c', 'qpoases3\src\Constraints.c', 'qpoases3\src\Indexlist.c', 'qpoases3\src\Matrices.c', 'qpoases3\src\MessageHandling.c', 'qpoases3\src\Options.c', 'qpoases3\src\Flipper.c', 'qpoases3\src\QProblem.c', 'qpoases3\src\QProblemB.c', 'qpoases3\src\Utils.c'};
      mask Help: <p>This block was generated automatically by the Legacy Code Tool. For detailed help on this tool, call<a href="matlab:legacy_code('help')"> legacy_code('help')</a>.</p>
      mask Callback ShowSpec:
      | if strcmp(get_param(gcbh, 'ShowSpec'), 'on')
      |   set_param(gcbh, 'MaskDisplay', sprintf('fprintf(''%s'');', get_param(gcbh, 'SFunctionSpec')));
      | else
      |   set_param(gcbh, 'MaskDisplay', sprintf('fprintf(''%s'');', get_param(gcbh, 'FunctionName')));
      | end
      mask Display: fprintf('acado_step(ACADOinput u1[1], ACADOoutput y1[1])');
  control : Constant  Value=0  OutDataTypeStr=int32
  initialization : Constant  Value=0  OutDataTypeStr=int32
  shifting : Constant  OutDataTypeStr=int32
  stage cost matrix : Constant  Value=reshape(diag([0 6e6 1e-4]),1,length(input.W)^2)
  terminal cost matrix : Constant  Value=reshape(diag([0 0]),1,length(input.WN)^2)
  Added yaw [Nm] : Outport
  wires:
  control/1 -> Bus Creator/1  "control"
  Bus Selector1/1 -> Selector/1  "<u>"
  initialization/1 -> Bus Creator/3  "initialization"
  acado_solver_sfun/1 -> Bus Selector1/1, Bus Assignment/1
  shifting/1 -> Bus Creator/2  "shifting"
  Bus Assignment/1 -> Bus Selector/1
  terminal cost matrix/1 -> Bus Assignment/6
  Initial conditions/1 -> Bus Assignment/4
  Shift reference/1(y) -> Bus Assignment/3
  stage cost matrix/1 -> Bus Assignment/5
  Bus Selector/1 -> Unit Delay/1  "<data>"
  Unit Delay/1 -> Bus Creator/4
  Bus Creator/1 -> acado_solver_sfun/1
  Selector/1 -> Added yaw [Nm]/1  "delta"
  Y/1 -> Shift reference/1(yN)
  X/1 -> Bus Assignment/2
  Shift reference2/1(y) -> Bus Assignment/7
  Vx/1 -> Shift reference2/1(yN)

== system MPC_Extended_Plant_Simulink/Case_2/Nonlinear Vehicle Model (9 DoF)1 ==
  steering wheel angle [rad] : Inport
  target pre-maneuver speed [m/s] : Inport  Port=2
  Add yaw moment [Nm] : Inport  Port=3
  Nonlinear Vehicle Model (9 DoF)_sfcn : S-Function  FunctionName=Nonlinear_sf  SFunctionModules=""  SFunctionDeploymentMode=off  EnableBusSupport=off  mask{rtw_sf_name=Nonlinear_sf, showVar=off}
      mask prompts: rtw_sf_name "Simulink:masks:GenSFuncName_MP"; showVar "Simulink:masks:GenSFuncShowModuleList_MP"
      mask help: Simulink:masks:GenSFuncDesc_MD
      mask init: same as MPC_Extended_Plant_Simulink/Case_1/Nonlinear Vehicle Model (9 DoF)/Nonlinear Vehicle Model (9 DoF)_sfcn
      settings: CopyFcn=|
      | if ~strcmp(get_param(gcb,'Linkstatus'),'none') && ...
      | ~strcmp(get_param(gcb,'Linkstatus'),'implicit')
      |   set_param(gcb,'LinkStatus','none');
      | end
      mask Help: eval('feval(''rtwprivate'',''rtwhelpview'',''rtw_sfcn_block'')');
      mask Display:
      | port_label('input',1,'steering wheel angle [rad]');
      | port_label('input',2,'target pre-maneuver speed [m/s]');
      | port_label('input',3,'Add yaw moment [Nm]');
      | port_label('output',1,'long velocity [m/s]');
      | port_label('output',2,'x-distance [m]');
      | port_label('output',3,'y-distance [m]');
      | port_label('output',4,'lat acceleration [m/s^2]');
      | port_label('output',5,'lat velocity [m/s]');
      | port_label('output',6,'yaw rate [rad/s]');
  __InputSSForSFun__ : Subsystem
  __OutputSSForSFun__ : Subsystem
  long velocity [m/s] : Outport  VectorParamsAs1DForOutWhenUnconnected=off
  x-distance [m] : Outport  Port=2  VectorParamsAs1DForOutWhenUnconnected=off
  y-distance [m] : Outport  Port=3  VectorParamsAs1DForOutWhenUnconnected=off
  lat acceleration [m/s^2] : Outport  Port=4  VectorParamsAs1DForOutWhenUnconnected=off
  lat velocity [m/s] : Outport  Port=5  VectorParamsAs1DForOutWhenUnconnected=off
  yaw rate [rad/s] : Outport  Port=6  VectorParamsAs1DForOutWhenUnconnected=off
  wires:
  steering wheel angle [rad]/1 -> __InputSSForSFun__/1(steering wheel angle [rad])
  target pre-maneuver speed [m/s]/1 -> __InputSSForSFun__/2(target pre-maneuver speed [m/s])
  __InputSSForSFun__/1(__UniqueOutportName__1__) -> Nonlinear Vehicle Model (9 DoF)_sfcn/1
  __InputSSForSFun__/3(__UniqueOutportName__3__) -> Nonlinear Vehicle Model (9 DoF)_sfcn/3
  Nonlinear Vehicle Model (9 DoF)_sfcn/1 -> __OutputSSForSFun__/1(__UniqueInportName__1__)
  Nonlinear Vehicle Model (9 DoF)_sfcn/2 -> __OutputSSForSFun__/2(__UniqueInportName__2__)
  Nonlinear Vehicle Model (9 DoF)_sfcn/3 -> __OutputSSForSFun__/3(__UniqueInportName__3__)
  Nonlinear Vehicle Model (9 DoF)_sfcn/4 -> __OutputSSForSFun__/4(__UniqueInportName__4__)
  Nonlinear Vehicle Model (9 DoF)_sfcn/5 -> __OutputSSForSFun__/5(__UniqueInportName__5__)
  Nonlinear Vehicle Model (9 DoF)_sfcn/6 -> __OutputSSForSFun__/6(__UniqueInportName__6__)
  __OutputSSForSFun__/1(long velocity [m/s]) -> long velocity [m/s]/1
  __OutputSSForSFun__/2(x-distance [m]) -> x-distance [m]/1
  __OutputSSForSFun__/3(y-distance [m]) -> y-distance [m]/1
  __OutputSSForSFun__/4(lat acceleration [m/s^2]) -> lat acceleration [m/s^2]/1
  __OutputSSForSFun__/5(lat velocity [m/s]) -> lat velocity [m/s]/1
  __OutputSSForSFun__/6(yaw rate [rad/s]) -> yaw rate [rad/s]/1
  __InputSSForSFun__/2(__UniqueOutportName__2__) -> Nonlinear Vehicle Model (9 DoF)_sfcn/2
  Add yaw moment [Nm]/1 -> __InputSSForSFun__/3(Add yaw moment [Nm])

== system MPC_Extended_Plant_Simulink/Case_2/Regerence Generator1 ==
  note: yawr_ref
  note: nonlinear response
  note: delta
  note: u
  steering wheel angle [rad] : Inport
  long velocity [m/s] : Inport  Port=2
  MATLAB Function : MATLAB Function  TreatAsAtomicUnit=on
  MATLAB Function1 : MATLAB Function  TreatAsAtomicUnit=on
  Transfer Fcn : TransferFcn  Numerator=[par.wn^2*par.tau par.wn^2]  Denominator=[1 2*par.kseta*par.wn par.wn^2]
  steering ratio : Gain  Gain=1/ par.i_steer
  reference yaw rate [rad/s] : Outport  VectorParamsAs1DForOutWhenUnconnected=off
  wires:
  steering wheel angle [rad]/1 -> steering ratio/1
  steering ratio/1 -> MATLAB Function/1(delta)
  long velocity [m/s]/1 -> MATLAB Function1/2(u), MATLAB Function/2(u)
  MATLAB Function/1(yawr_ss) -> MATLAB Function1/1(yawr_ss)
  MATLAB Function1/1(yawr_sat) -> Transfer Fcn/1
  Transfer Fcn/1 -> reference yaw rate [rad/s]/1

== system MPC_Extended_Plant_Simulink/Case_3/Driver: Sine with Dwell2 ==
  Constant1 : Constant
  Lookup Table1 : Lookup  InputValues=[0:0.1:3*pi/2 3*pi/2+eps]*0.7  Table=sin([0:0.1:3*pi/2 3*pi/2+eps])  LookUpMeth=Interpolation-Use End Values  SaturateOnIntegerOverflow=off
  Lookup Table2 : Lookup  InputValues=[3*pi/2:0.1:2*pi 2*pi+eps]*0.7  Table=sin([3*pi/2:0.1:2*pi 2*pi+eps])  LookUpMeth=Interpolation-Use End Values  SaturateOnIntegerOverflow=off
  Ramp6 : simulink/Sources/Ramp  slope=pi  start=10  InitialOutput=0
  Ramp7 : simulink/Sources/Ramp  slope=pi  start=10+0.5  InitialOutput=0
  Subtract1 : Sum  Inputs=+++
  amplitude : Gain  Gain=120
  deg2rad : Gain  Gain=pi / 180
  steering wheel angle [rad] : Outport  VectorParamsAs1DForOutWhenUnconnected=off
  wires:
  Ramp6/1 -> Lookup Table1/1
  Ramp7/1 -> Lookup Table2/1
  Lookup Table2/1 -> Subtract1/2
  Lookup Table1/1 -> Subtract1/1
  Constant1/1 -> Subtract1/3
  Subtract1/1 -> amplitude/1
  amplitude/1 -> deg2rad/1
  deg2rad/1 -> steering wheel angle [rad]/1

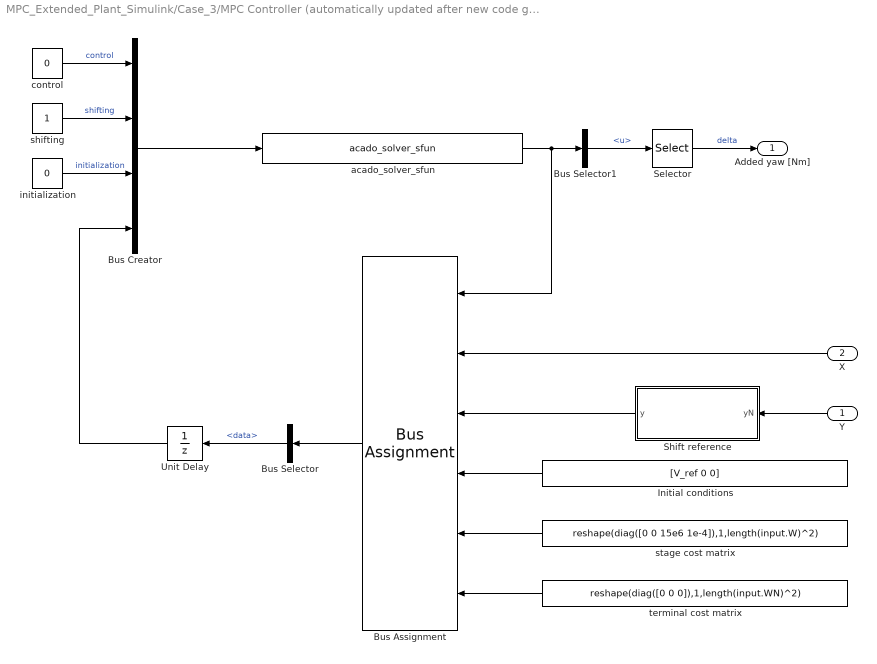
== system MPC_Extended_Plant_Simulink/Case_3/MPC Controller (automatically updated after new code generation)2 ==
  Y : Inport
  X : Inport  Port=2
  Bus Assignment : BusAssignment  AssignedSignals=data.x0,data.y,data.yN,data.W,data.WN
  Bus Creator : BusCreator  Inputs=4  OutDataTypeStr=Bus: ACADOinput
  Bus Selector : BusSelector  OutputSignals=data
  Bus Selector1 : BusSelector  OutputSignals=data.u
  Initial conditions : Constant  Value=[V_ref 0 0]
  Selector : Selector  InputPortWidth=Np  IndexOptions=Starting index (dialog)  Indices=[1]  OutputSizes=1
  Shift reference : MATLAB Function  TreatAsAtomicUnit=on
  Unit Delay : UnitDelay  InitialCondition=init  SampleTime=Ts  HasFrameUpgradeWarning=on
  acado_solver_sfun : S-Function  FunctionName=acado_solver_sfun  SFunctionDeploymentMode=off  EnableBusSupport=off  mask(Legacy Function){SFunctionSpec=acado_step(ACADOinput u1[1], ACADOoutput y1[1]), ShowSpec=on}
      mask prompts: ShowSpec "Display function specification"
      mask help:
      | This block allows you to call the legacy functions specified by the following Legacy Code Tool definition:
      | def.SFunctionName = 'acado_solver_sfun';
      | def.OutputFcnSpec = 'acado_step(ACADOinput u1[1], ACADOoutput y1[1])';
      | def.StartFcnSpec = 'acado_initialize( void )';
      | def.TerminateFcnSpec = 'acado_cleanup( void )';
      | def.HeaderFiles = {'acado_common.h', 'acado_solver_sfunction.h'};
      | def.SourceFiles = {'acado_solver.c', 'acado_integrator.c', 'acado_auxiliary_functions.c', 'acado_solver_sfunction.c', 'acado_qpoases3_interface.c', 'qpoases3\src\Bounds.c', 'qpoases3\src\Constraints.c', 'qpoases3\src\Indexlist.c', 'qpoases3\src\Matrices.c', 'qpoases3\src\MessageHandling.c', 'qpoases3\src\Options.c', 'qpoases3\src\Flipper.c', 'qpoases3\src\QProblem.c', 'qpoases3\src\QProblemB.c', 'qpoases3\src\Utils.c'};
      mask Help: <p>This block was generated automatically by the Legacy Code Tool. For detailed help on this tool, call<a href="matlab:legacy_code('help')"> legacy_code('help')</a>.</p>
      mask Callback ShowSpec:
      | if strcmp(get_param(gcbh, 'ShowSpec'), 'on')
      |   set_param(gcbh, 'MaskDisplay', sprintf('fprintf(''%s'');', get_param(gcbh, 'SFunctionSpec')));
      | else
      |   set_param(gcbh, 'MaskDisplay', sprintf('fprintf(''%s'');', get_param(gcbh, 'FunctionName')));
      | end
      mask Display: fprintf('acado_step(ACADOinput u1[1], ACADOoutput y1[1])');
  control : Constant  Value=0  OutDataTypeStr=int32
  initialization : Constant  Value=0  OutDataTypeStr=int32
  shifting : Constant  OutDataTypeStr=int32
  stage cost matrix : Constant  Value=reshape(diag([0 0 15e6 1e-4]),1,length(input.W)^2)
  terminal cost matrix : Constant  Value=reshape(diag([0 0 0]),1,length(input.WN)^2)
  Added yaw [Nm] : Outport
  wires:
  control/1 -> Bus Creator/1  "control"
  Bus Selector1/1 -> Selector/1  "<u>"
  initialization/1 -> Bus Creator/3  "initialization"
  acado_solver_sfun/1 -> Bus Selector1/1, Bus Assignment/1
  shifting/1 -> Bus Creator/2  "shifting"
  Bus Assignment/1 -> Bus Selector/1
  terminal cost matrix/1 -> Bus Assignment/6
  Initial conditions/1 -> Bus Assignment/4
  Shift reference/1(y) -> Bus Assignment/3
  stage cost matrix/1 -> Bus Assignment/5
  Bus Selector/1 -> Unit Delay/1  "<data>"
  Unit Delay/1 -> Bus Creator/4
  Bus Creator/1 -> acado_solver_sfun/1
  Selector/1 -> Added yaw [Nm]/1  "delta"
  Y/1 -> Shift reference/1(yN)
  X/1 -> Bus Assignment/2

== system MPC_Extended_Plant_Simulink/Case_3/Nonlinear Vehicle Model (9 DoF)2 ==
  steering wheel angle [rad] : Inport
  target pre-maneuver speed [m/s] : Inport  Port=2
  Add yaw moment [Nm] : Inport  Port=3
  Nonlinear Vehicle Model (9 DoF)_sfcn : S-Function  FunctionName=Nonlinear_sf  SFunctionModules=""  SFunctionDeploymentMode=off  EnableBusSupport=off  mask{rtw_sf_name=Nonlinear_sf, showVar=off}
      mask prompts: rtw_sf_name "Simulink:masks:GenSFuncName_MP"; showVar "Simulink:masks:GenSFuncShowModuleList_MP"
      mask help: Simulink:masks:GenSFuncDesc_MD
      mask init: same as MPC_Extended_Plant_Simulink/Case_1/Nonlinear Vehicle Model (9 DoF)/Nonlinear Vehicle Model (9 DoF)_sfcn
      settings: CopyFcn=|
      | if ~strcmp(get_param(gcb,'Linkstatus'),'none') && ...
      | ~strcmp(get_param(gcb,'Linkstatus'),'implicit')
      |   set_param(gcb,'LinkStatus','none');
      | end
      mask Help: eval('feval(''rtwprivate'',''rtwhelpview'',''rtw_sfcn_block'')');
      mask Display:
      | port_label('input',1,'steering wheel angle [rad]');
      | port_label('input',2,'target pre-maneuver speed [m/s]');
      | port_label('input',3,'Add yaw moment [Nm]');
      | port_label('output',1,'long velocity [m/s]');
      | port_label('output',2,'x-distance [m]');
      | port_label('output',3,'y-distance [m]');
      | port_label('output',4,'lat acceleration [m/s^2]');
      | port_label('output',5,'lat velocity [m/s]');
      | port_label('output',6,'yaw rate [rad/s]');
  __InputSSForSFun__ : Subsystem
  __OutputSSForSFun__ : Subsystem
  long velocity [m/s] : Outport  VectorParamsAs1DForOutWhenUnconnected=off
  x-distance [m] : Outport  Port=2  VectorParamsAs1DForOutWhenUnconnected=off
  y-distance [m] : Outport  Port=3  VectorParamsAs1DForOutWhenUnconnected=off
  lat acceleration [m/s^2] : Outport  Port=4  VectorParamsAs1DForOutWhenUnconnected=off
  lat velocity [m/s] : Outport  Port=5  VectorParamsAs1DForOutWhenUnconnected=off
  yaw rate [rad/s] : Outport  Port=6  VectorParamsAs1DForOutWhenUnconnected=off
  wires:
  steering wheel angle [rad]/1 -> __InputSSForSFun__/1(steering wheel angle [rad])
  target pre-maneuver speed [m/s]/1 -> __InputSSForSFun__/2(target pre-maneuver speed [m/s])
  __InputSSForSFun__/1(__UniqueOutportName__1__) -> Nonlinear Vehicle Model (9 DoF)_sfcn/1
  __InputSSForSFun__/3(__UniqueOutportName__3__) -> Nonlinear Vehicle Model (9 DoF)_sfcn/3
  Nonlinear Vehicle Model (9 DoF)_sfcn/1 -> __OutputSSForSFun__/1(__UniqueInportName__1__)
  Nonlinear Vehicle Model (9 DoF)_sfcn/2 -> __OutputSSForSFun__/2(__UniqueInportName__2__)
  Nonlinear Vehicle Model (9 DoF)_sfcn/3 -> __OutputSSForSFun__/3(__UniqueInportName__3__)
  Nonlinear Vehicle Model (9 DoF)_sfcn/4 -> __OutputSSForSFun__/4(__UniqueInportName__4__)
  Nonlinear Vehicle Model (9 DoF)_sfcn/5 -> __OutputSSForSFun__/5(__UniqueInportName__5__)
  Nonlinear Vehicle Model (9 DoF)_sfcn/6 -> __OutputSSForSFun__/6(__UniqueInportName__6__)
  __OutputSSForSFun__/1(long velocity [m/s]) -> long velocity [m/s]/1
  __OutputSSForSFun__/2(x-distance [m]) -> x-distance [m]/1
  __OutputSSForSFun__/3(y-distance [m]) -> y-distance [m]/1
  __OutputSSForSFun__/4(lat acceleration [m/s^2]) -> lat acceleration [m/s^2]/1
  __OutputSSForSFun__/5(lat velocity [m/s]) -> lat velocity [m/s]/1
  __OutputSSForSFun__/6(yaw rate [rad/s]) -> yaw rate [rad/s]/1
  __InputSSForSFun__/2(__UniqueOutportName__2__) -> Nonlinear Vehicle Model (9 DoF)_sfcn/2
  Add yaw moment [Nm]/1 -> __InputSSForSFun__/3(Add yaw moment [Nm])

== system MPC_Extended_Plant_Simulink/Case_3/Regerence Generator2 ==
  note: yawr_ref
  note: nonlinear response
  note: delta
  note: u
  steering wheel angle [rad] : Inport
  long velocity [m/s] : Inport  Port=2
  MATLAB Function : MATLAB Function  TreatAsAtomicUnit=on
  MATLAB Function1 : MATLAB Function  TreatAsAtomicUnit=on
  Transfer Fcn : TransferFcn  Numerator=[par.wn^2*par.tau par.wn^2]  Denominator=[1 2*par.kseta*par.wn par.wn^2]
  steering ratio : Gain  Gain=1/ par.i_steer
  reference yaw rate [rad/s] : Outport  VectorParamsAs1DForOutWhenUnconnected=off
  wires:
  steering wheel angle [rad]/1 -> steering ratio/1
  steering ratio/1 -> MATLAB Function/1(delta)
  long velocity [m/s]/1 -> MATLAB Function1/2(u), MATLAB Function/2(u)
  MATLAB Function/1(yawr_ss) -> MATLAB Function1/1(yawr_ss)
  MATLAB Function1/1(yawr_sat) -> Transfer Fcn/1
  Transfer Fcn/1 -> reference yaw rate [rad/s]/1

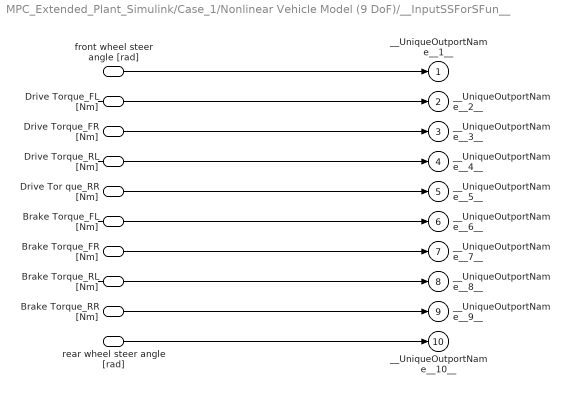
== system MPC_Extended_Plant_Simulink/Case_1/Nonlinear Vehicle Model (9 DoF)/__InputSSForSFun__ ==
  front wheel steer angle [rad] : Inport
  Drive Torque_FL [Nm] : Inport  Port=2
  Drive Torque_FR [Nm] : Inport  Port=3
  Drive Torque_RL [Nm] : Inport  Port=4
  Drive Tor	que_RR [Nm] : Inport  Port=5
  Brake Torque_FL [Nm] : Inport  Port=6
  Brake Torque_FR [Nm] : Inport  Port=7
  Brake Torque_RL [Nm] : Inport  Port=8
  Brake Torque_RR [Nm] : Inport  Port=9
  rear wheel steer angle [rad] : Inport  Port=10
  __UniqueOutportName__1__ : Outport
  __UniqueOutportName__2__ : Outport  Port=2
  __UniqueOutportName__3__ : Outport  Port=3
  __UniqueOutportName__4__ : Outport  Port=4
  __UniqueOutportName__5__ : Outport  Port=5
  __UniqueOutportName__6__ : Outport  Port=6
  __UniqueOutportName__7__ : Outport  Port=7
  __UniqueOutportName__8__ : Outport  Port=8
  __UniqueOutportName__9__ : Outport  Port=9
  __UniqueOutportName__10__ : Outport  Port=10
  wires:
  front wheel steer angle [rad]/1 -> __UniqueOutportName__1__/1
  Drive Torque_FL [Nm]/1 -> __UniqueOutportName__2__/1
  Drive Torque_FR [Nm]/1 -> __UniqueOutportName__3__/1
  Drive Torque_RL [Nm]/1 -> __UniqueOutportName__4__/1
  Drive Tor	que_RR [Nm]/1 -> __UniqueOutportName__5__/1
  Brake Torque_FL [Nm]/1 -> __UniqueOutportName__6__/1
  Brake Torque_FR [Nm]/1 -> __UniqueOutportName__7__/1
  Brake Torque_RL [Nm]/1 -> __UniqueOutportName__8__/1
  Brake Torque_RR [Nm]/1 -> __UniqueOutportName__9__/1
  rear wheel steer angle [rad]/1 -> __UniqueOutportName__10__/1

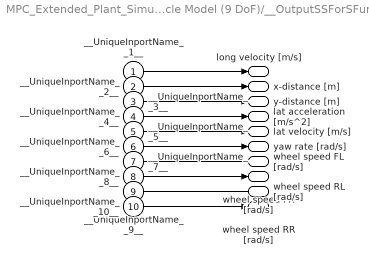
== system MPC_Extended_Plant_Simulink/Case_1/Nonlinear Vehicle Model (9 DoF)/__OutputSSForSFun__ ==
  __UniqueInportName__1__ : Inport
  __UniqueInportName__2__ : Inport  Port=2
  __UniqueInportName__3__ : Inport  Port=3
  __UniqueInportName__4__ : Inport  Port=4
  __UniqueInportName__5__ : Inport  Port=5
  __UniqueInportName__6__ : Inport  Port=6
  __UniqueInportName__7__ : Inport  Port=7
  __UniqueInportName__8__ : Inport  Port=8
  __UniqueInportName__9__ : Inport  Port=9
  __UniqueInportName__10__ : Inport  Port=10
  long velocity [m/s] : Outport  VectorParamsAs1DForOutWhenUnconnected=off
  x-distance [m] : Outport  Port=2  VectorParamsAs1DForOutWhenUnconnected=off
  y-distance [m] : Outport  Port=3  VectorParamsAs1DForOutWhenUnconnected=off
  lat acceleration [m/s^2] : Outport  Port=4  VectorParamsAs1DForOutWhenUnconnected=off
  lat velocity [m/s] : Outport  Port=5  VectorParamsAs1DForOutWhenUnconnected=off
  yaw rate [rad/s] : Outport  Port=6  VectorParamsAs1DForOutWhenUnconnected=off
  wheel speed FL [rad/s] : Outport  Port=7  VectorParamsAs1DForOutWhenUnconnected=off
  wheel speed FR [rad/s] : Outport  Port=8  VectorParamsAs1DForOutWhenUnconnected=off
  wheel speed RL [rad/s] : Outport  Port=9  VectorParamsAs1DForOutWhenUnconnected=off
  wheel speed RR [rad/s] : Outport  Port=10  VectorParamsAs1DForOutWhenUnconnected=off
  wires:
  __UniqueInportName__1__/1 -> long velocity [m/s]/1
  __UniqueInportName__2__/1 -> x-distance [m]/1
  __UniqueInportName__3__/1 -> y-distance [m]/1
  __UniqueInportName__4__/1 -> lat acceleration [m/s^2]/1
  __UniqueInportName__5__/1 -> lat velocity [m/s]/1
  __UniqueInportName__6__/1 -> yaw rate [rad/s]/1
  __UniqueInportName__7__/1 -> wheel speed FL [rad/s]/1
  __UniqueInportName__8__/1 -> wheel speed FR [rad/s]/1
  __UniqueInportName__9__/1 -> wheel speed RL [rad/s]/1
  __UniqueInportName__10__/1 -> wheel speed RR [rad/s]/1

== system MPC_Extended_Plant_Simulink/Case_2/Nonlinear Vehicle Model (9 DoF)1/__InputSSForSFun__ ==
  steering wheel angle [rad] : Inport
  target pre-maneuver speed [m/s] : Inport  Port=2
  Add yaw moment [Nm] : Inport  Port=3
  __UniqueOutportName__1__ : Outport
  __UniqueOutportName__2__ : Outport  Port=2
  __UniqueOutportName__3__ : Outport  Port=3
  wires:
  steering wheel angle [rad]/1 -> __UniqueOutportName__1__/1
  target pre-maneuver speed [m/s]/1 -> __UniqueOutportName__2__/1
  Add yaw moment [Nm]/1 -> __UniqueOutportName__3__/1
